simulink model "tutorial_simulink_3"  (R2024b)
settings: Solver=VariableStepAuto  StartTime=0.0  StopTime=10.0  RelTol=1e-3
settings Model: Creator=俞书阳  LastModifiedBy=user

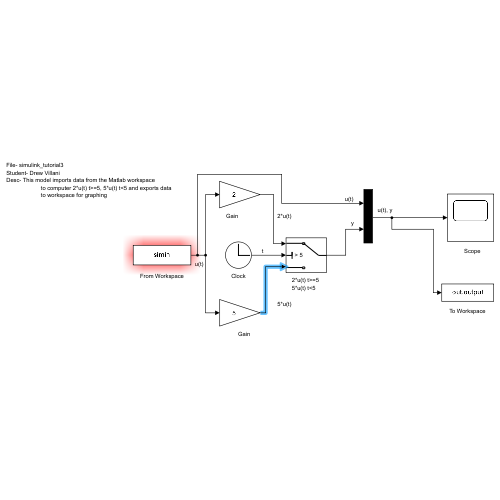
[thumbnail: Simulink's stored preview of the top-level diagram]
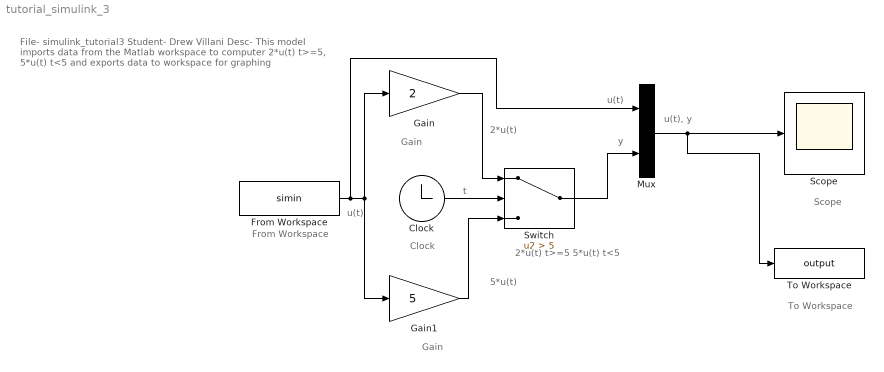
== system tutorial_simulink_3 ==
  note: File- simulink_tutorial3
      | Student- Drew Villani
      | Desc- This model imports data from the Matlab workspace
      | 			to computer 2*u(t) t>=5, 5*u(t) t<5 and exports data
      | 			to workspace for graphing
  note: To Workspace
  note: Scope
  note: u(t), y
  note: u(t)
  note: y
  note: 2*u(t) t>=5
      | 5*u(t) t<5
  note: 5*u(t)
  note: 2*u(t)
  note: Gain
  note: Gain
  note: t
  note: Clock
  note: u(t)
  note: From Workspace
  Clock : Clock
  From Workspace : FromWorkspace  VariableName=simin
  Gain : Gain  Gain=2
  Gain1 : Gain  Gain=5
  Mux : Mux  Inputs=2
  Scope : Scope
  Switch : Switch  Criteria=u2 > Threshold  Threshold=5  SaturateOnIntegerOverflow=off  InputSameDT=off
  To Workspace : ToWorkspace  VariableName=output  SaveFormat=Timeseries  SampleTime=-1
  wires:
  Clock/1 -> Switch/2
  Gain/1 -> Switch/1
  Gain1/1 -> Switch/3
  From Workspace/1 -> Mux/1, Gain1/1, Gain/1
  Mux/1 -> To Workspace/1, Scope/1
  Switch/1 -> Mux/2
